simulink model "Simulink"  (R2025b)
settings: Solver=FixedStepDiscrete  StartTime=0.0  StopTime=inf  RelTol=1e-3
settings Model: Creator=hassa  LastModifiedBy=hassa
settings OptimizationCC: DefaultParameterBehavior=Inlined  UseDivisionForNetSlopeComputation=on  GainParamInheritBuiltInType=on  UseFloatMulNetSlope=on  InlineInvariantSignals=on  PassReuseOutputArgsAs=Individual arguments  ZeroExternalMemoryAtStartup=off  ZeroInternalMemoryAtStartup=off  NoFixptDivByZeroProtection=on  EfficientFloat2IntCast=on  LifeSpan=1  MaxStackSize=512  OptimizeBlockOrder=speed  DifferentSizesBufferReuse=on  EfficientTunableParamExpr=on
settings DebuggingCC: ParameterTunabilityLossMsg=error
settings HardwareCC: ProdBitPerPointer=32.0  ProdBitPerSizeT=32.0  ProdBitPerPtrDiffT=32.0  ProdLargestAtomicInteger=Long  ProdLargestAtomicFloat=Double  ProdWordSize=32.0  ProdLongLongMode=on  ProdHWDeviceType=ARM Compatible->ARM Cortex-M
settings SFSimCC: MATLABDynamicMemAlloc=off
settings RTWCC: SystemTargetFile=ert.tlc  HardwareBoard=STM32H7xx Based (Single-core)  TemplateMakefile=ert_default_tmf  Toolchain=GNU Tools for ARM Embedded Processors  Description=Embedded Coder
settings CodeAppCC: ForceParamTrailComments=on  IgnoreCustomStorageClasses=off  OperatorAnnotations=on  SimulinkDataObjDesc=on  SFDataObjDesc=on  CustomSymbolStrGlobalVar=rt$N$M  CustomSymbolStrType=$N$M  CustomSymbolStrFcn=$N$M$F  CustomSymbolStrMacro=$N$M  InsertBlockDesc=on
settings ERTTargetCC: ExtModeTransport=3.0  ExtModeStaticAlloc=on  ExtModeStaticAllocSize=2048.0  ExtModeMexFile=ext_xcp  ExtModeIntrfLevel=Level2 - Open  ERTFilePackagingFormat=CompactWithDataFile  TargetLangStandard=C99 (ISO)  CodeReplacementLibrary=ARM Cortex-M  IncludeMdlTerminateFcn=off  CombineSignalStateStructs=on  SupportAbsoluteTime=off  SupportComplex=off  SupportNonInlinedSFcns=on

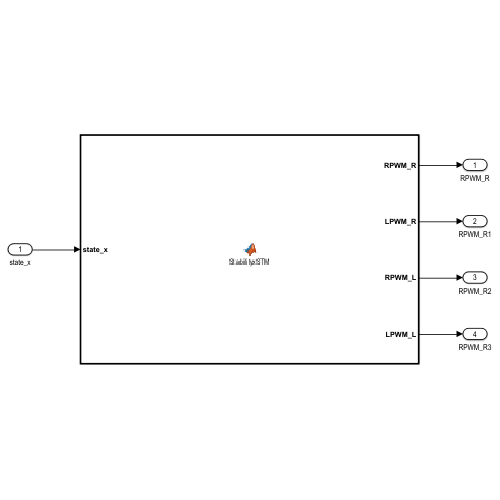
[thumbnail: Simulink's stored preview of the top-level diagram]
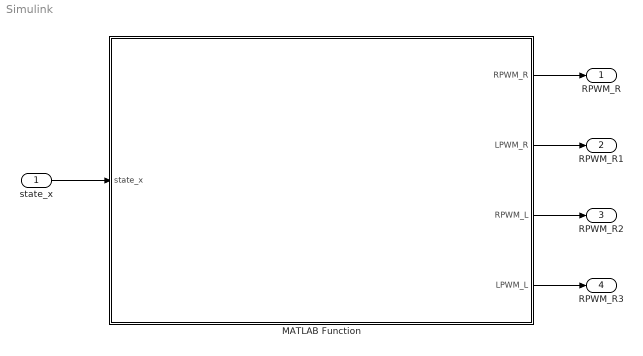
== system Simulink ==
  state_x : Inport  PortDimensions=[6,1]
  MATLAB Function : MATLAB Function  TreatAsAtomicUnit=on
  RPWM_R : Outport
  RPWM_R1 : Outport  Port=2
  RPWM_R2 : Outport  Port=3
  RPWM_R3 : Outport  Port=4
  wires:
  state_x/1 -> MATLAB Function/1(state_x)
  MATLAB Function/1(RPWM_R) -> RPWM_R/1
  MATLAB Function/2(LPWM_R) -> RPWM_R1/1
  MATLAB Function/3(RPWM_L) -> RPWM_R2/1
  MATLAB Function/4(LPWM_L) -> RPWM_R3/1

== matlab function Simulink/MATLAB Function ==
  data: state_x input; RPWM_R output; LPWM_R output; RPWM_L output; LPWM_L output
function [RPWM_R, LPWM_R, RPWM_L, LPWM_L] = StabilityxSTM(state_x)
    %#codegen
    % Real-time LQR controller for Wheel-Biped Robot on STM32
    %
    % Inputs:
    %   state_x  : 6x1 state vector [phi; s; theta; phi_dot; v; omega]
    % Outputs:
    %   RPWM_R, LPWM_R : Right motor PWM signals (0 to 1000)
    %   RPWM_L, LPWM_L : Left motor PWM signals (0 to 1000)
    
    % 1. System Constants
    V_batt = 24.0;
    max_pwm = 1000;
    
    % Define the pre-computed K matrix using standard MATLAB syntax.
    % Simulink Coder will automatically convert this into a constant C array.
    K_matrix = [-12.4395, -0.7071,  0.7071, -2.9489, -1.3601,  0.7289;
                -12.4395, -0.7071, -0.7071, -2.9489, -1.3601, -0.7289];

    % 2. Calculate Control Effort (u = -K * x)
    % The output u will be a 2x1 vector [tau_r; tau_l]. 
    % We treat these commanded torques as commanded voltages (v_r, v_l) 
    % for the motor driver mapping.
    u = -K_matrix * state_x;
    
    v_r = u(1);
    v_l = u(2);
    
    % 3. Convert to PWM and Clamp
    pwm_r = round((v_r / V_batt) * max_pwm);
    pwm_l = round((v_l / V_batt) * max_pwm);
    
    % Clamping logic
    pwm_r = max(min(pwm_r, max_pwm), -max_pwm);
    pwm_l = max(min(pwm_l, max_pwm), -max_pwm);
    
    % 4. Directional Splitting for Right Motor
    if pwm_r >= 0
        RPWM_R = pwm_r;
        LPWM_R = 0;
    else
        RPWM_R = 0;
        LPWM_R = abs(pwm_r); 
    end
    
    % 5. Directional Splitting for Left Motor
    if pwm_l >= 0
        RPWM_L = pwm_l;
        LPWM_L = 0;
    else
        RPWM_L = 0;
        LPWM_L = abs(pwm_l); 
    end
end
